simulink model "Controller_Simulation"  (R2025b)
settings: Solver=VariableStepAuto  StartTime=0.0  StopTime=100  RelTol=1e-3
undefined symbols (not defined in the file): cg_structure, chi, DiscIntNeverNeededParam, ESC_mass_same, g, Kd, Ki, Kp, M, m_carriage_bracket_and_cart, m_counter, m_struct, miu_k, Motor_mass_small, N, prop_mass_small
libraries: simulink x3, slpidlib x1, SignalEditorBlockLib x1
settings Model: Creator=adity  LastModifiedBy=33248

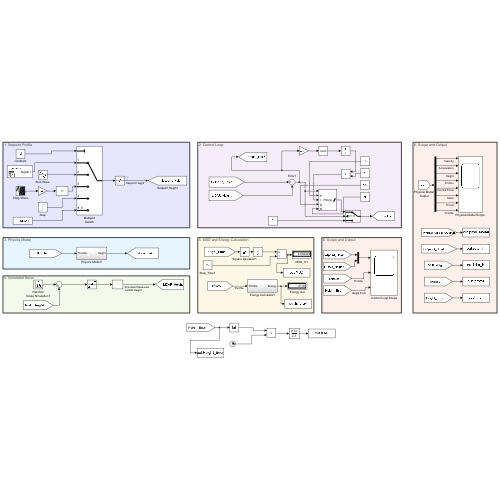
[thumbnail: Simulink's stored preview of the top-level diagram]
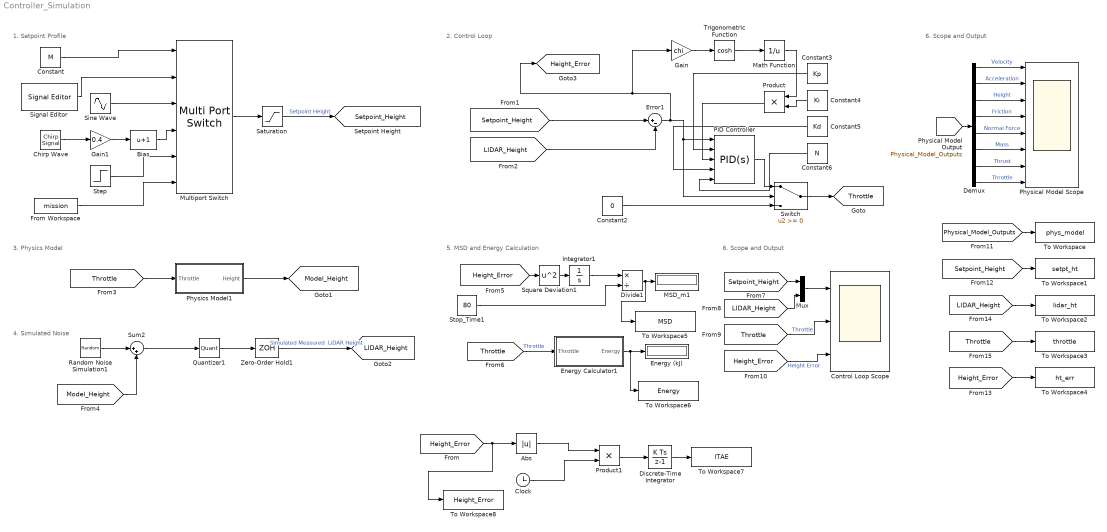
== system Controller_Simulation ==
  note: 6. Scope and Output
  note: 6. Scope and Output
  note: 5. MSD and Energy Calculation
  note: 4. Simulated Noise
  note: 3. Physics Model
  note: 2. Control Loop
  note: 1. Setpoint Profile
  Abs : Abs  SaturateOnIntegerOverflow=off
  Bias : Bias  Bias=1  SaturateOnIntegerOverflow=off
  Chirp Wave : simulink/Sources/Chirp Signal  f1=0.01  T=100  f2=0.5
  Clock : Clock
  Constant : Constant  Value=M
  Constant2 : Constant  Value=0
  Constant3 : Constant  Value=Kp
  Constant4 : Constant  Value=Ki
  Constant5 : Constant  Value=Kd
  Constant6 : Constant  Value=N
  Control Loop Scope : Scope  NumInputPorts=3
      settings: ActiveDisplayYMinimum=-0.74940462387190931  ActiveDisplayYMaximum=2.1498858123443716  DataLoggingVariableName=ScopeData2
  Demux : Demux  Outputs=8
  Discrete-Time Integrator : DiscreteIntegrator  SampleTime=-1  ICPrevOutput=DiscIntNeverNeededParam  ICPrevScaledInput=DiscIntNeverNeededParam
  Divide1 : Product  Inputs=*/
  Energy (kJ) : Display
  Energy Calculator1 : Subsystem
  Error1 : Sum  Inputs=|+-
  From Workspace : FromWorkspace  VariableName=mission
  Gain : Gain  Gain=chi
  Gain1 : Gain  Gain=0.4
  Integrator1 : Integrator
  MSD_m1 : Display
  Math Function : Math  Operator=reciprocal
  Multiport Switch : MultiPortSwitch  Inputs=5  SaturateOnIntegerOverflow=off  InputSameDT=off
  Mux : Mux  Inputs=2
  PID Controller : slpidlib/PID Controller  Controller=PID  Form=Parallel  TimeDomain=Continuous-time  UseExternalTs=off  SampleTime=-1  IntegratorMethod=Forward Euler  FilterMethod=Forward Euler  ControllerParametersSource=external  P=230  I=75  UseKiTs=off  D=50  UseExternalDerivativeSource=off  N=10  UseFilter=on  TunerSelectOption=Transfer Function Based (PID Tuner App)  InitialConditionSource=internal  InitialConditionForIntegrator=0  InitialConditionForFilter=0  DifferentiatorICPrevScaledInput=0  ExternalReset=none  TrackingMode=off  Kt=1  LimitOutput=on  SatLimitsSource=internal  UpperSaturationLimit=79.0425  LowerSaturationLimit=0  LinearizeAsGain=on  AntiWindupMode=clamping  Kb=1  LimitIntegrator=off  UpperIntegratorSaturationLimit=inf  LowerIntegratorSaturationLimit=-inf  POutMin=[]  POutMax=[]  IOutMin=[]  IOutMax=[]  DOutMin=[]  DOutMax=[]  NOutMin=[]  NOutMax=[]  SumOutMin=[]  SumOutMax=[]  SaturationOutMin=[]  SaturationOutMax=[]  PParamMin=[]  PParamMax=[]  IParamMin=[]  IParamMax=[]  DParamMin=[]  DParamMax=[]  NParamMin=[]  NParamMax=[]  KbParamMin=[]  KbParamMax=[]  KtParamMin=[]  KtParamMax=[]  KbOutMin=[]  KbOutMax=[]  KtOutMin=[]  KtOutMax=[]  IntegratorOutMin=[]  IntegratorOutMax=[]  FilterOutMin=[]  FilterOutMax=[]  SumI1OutMin=[]  SumI1OutMax=[]  SumI2OutMin=[]  SumI2OutMax=[]  SumI3OutMin=[]  SumI3OutMax=[]  SumI4OutMin=[]  SumI4OutMax=[]  SumDOutMin=[]  SumDOutMax=[]  DifferentiatorOutMin=[]  DifferentiatorOutMax=[]  FilterDiffOutCoefMin=[]  FilterDiffOutCoefMax=[]  ReciprocalOutMin=[]  ReciprocalOutMax=[]  SumDenOutMin=[]  SumDenOutMax=[]  SumNumOutMin=[]  SumNumOutMax=[]  DivideOutMin=[]  DivideOutMax=[]  UdiffTsProdOutMin=[]  UdiffTsProdOutMax=[]  NTsProdOutMin=[]  NTsProdOutMax=[]  UintegralTsProdOutMin=[]  UintegralTsProdOutMax=[]  UngainTsProdOutMin=[]  UngainTsProdOutMax=[]  ClampingZeroOutDataTypeStr=Inherit: Inherit via back propagation  ClampingZeroOutMin=[]  ClampingZeroOutMax=[]  FilterDenConstantOutDataTypeStr=Inherit: Inherit via back propagation  FilterDenConstantOutMin=[]  FilterDenConstantOutMax=[]  PCopyOutDataTypeStr=Inherit: Inherit via back propagation  PCopyOutMin=[]  PCopyOutMax=[]  NCopyOutDataTypeStr=Inherit: Inherit via back propagation  NCopyOutMin=[]  NCopyOutMax=[]  IntegratorContinuousStateAttributes=''  IntegratorStateMustResolveToSignalObject=off  IntegratorRTWStateStorageClass=Auto  FilterContinuousStateAttributes=''  FilterStateMustResolveToSignalObject=off  FilterRTWStateStorageClass=Auto  ParallelPVariant=ExternalParameters  IdealPVariant=Disabled  IVariant=ExternalParameters  DVariant=ExternalParameters  IntegratorVariant=Continuous  SatVariant=Enabled  AWVariant=ContClampingParallel  PCopyVariant=Disabled  TRVariant=Disabled  FdbkBlocksVariant=Forward  IdealPFdbkVariant=Disabled  SatFdbkVariant=Disabled  DerivativeFilterVariant=ContFilter  NVariant=ExternalParameters  NCopyVariant=Disabled  FilterICVariant=InternalICsFilter  IntegratorICVariant=InternalICs  ExternalResetVariant=Disabled  TRSumVariant=Passthrough  SumFdbkVariant=Disabled  SumVariant=Sum_PID  TsampFilterVariant=InternalTs  TsampNgainVariant=Passthrough  TsampIntegralVariant=Disabled_SignalSpec  ExternalSaturationOutDataTypeStr=Inherit: Same as second input  DerivativeSourceVariant=ErrorSignal  PreIntVariant=InternalPreInt
  Physical Model Scope : Scope  NumInputPorts=8
      settings: ActiveDisplayYMinimum=0.51277748941499457  ActiveDisplayYMaximum=1.1096551033755411  DataLoggingVariableName=ScopeData3
  Physics Model1 : Subsystem
  Product : Product
  Product1 : Product
  Quantizer1 : Quantizer  QuantizationInterval=0.001
  Random Noise Simulation1 : RandomNumber  Variance=5e-05  SampleTime=0.05
  Saturation : Saturate  UpperLimit=1.44  LowerLimit=0
  Signal Editor : SignalEditorBlockLib/Signal Editor  FileName=samplemission.mat  ActiveScenario=Scenario  ActiveSignal=Signal 1  IsBus=off  OutputBusObjectStr=Bus: BusObject  SampleTime=0  ZeroCross=off  OutputAfterFinalValue=Setting to zero  Unit=inherit  PreserveSignalName=on  ApplySigPropsToAllScenarios=on  ApplySigPropsToAllSignals=off  SignalPropertySource=Dialog parameters
  Sine Wave : Sin  Amplitude=1.44  SampleTime=0
  Square Deviation1 : Math  Operator=square
  Step : Step  Time=20  After=1.3  SampleTime=0
  Stop_Time1 : Constant  Value=80
  Sum2 : Sum  Inputs=|++
  Switch : Switch  SaturateOnIntegerOverflow=off  InputSameDT=off
  To Workspace : ToWorkspace  VariableName=phys_model  SaveFormat=Timeseries  SampleTime=-1
  To Workspace1 : ToWorkspace  VariableName=setpt_ht  SaveFormat=Timeseries  SampleTime=-1
  To Workspace2 : ToWorkspace  VariableName=lidar_ht  SaveFormat=Timeseries  SampleTime=-1
  To Workspace3 : ToWorkspace  VariableName=throttle  SaveFormat=Timeseries  SampleTime=-1
  To Workspace4 : ToWorkspace  VariableName=ht_err  SaveFormat=Timeseries  SampleTime=-1
  To Workspace5 : ToWorkspace  VariableName=MSD  SaveFormat=Timeseries  SampleTime=-1
  To Workspace6 : ToWorkspace  VariableName=Energy  SaveFormat=Timeseries  SampleTime=-1
  To Workspace7 : ToWorkspace  VariableName=ITAE  SaveFormat=Timeseries  SampleTime=-1
  To Workspace8 : ToWorkspace  VariableName=Height_Error  SaveFormat=Timeseries  SampleTime=-1
  Trigonometric Function : Trigonometry  Operator=cosh
  Zero-Order Hold1 : ZeroOrderHold  SampleTime=0.05
  tag scope: Height_Error=global, LIDAR_Height=global, Model_Height=global, Setpoint_Height=global, Throttle=global
  wires:
  Step/1 -> Multiport Switch/5
  Constant/1 -> Multiport Switch/1
  Multiport Switch/1 -> Saturation/1
  Saturation/1 -> [Setpoint_Height]  "Setpoint Height"
  Sine Wave/1 -> Multiport Switch/3
  [LIDAR_Height] -> Error1/2
  PID Controller/1 -> Switch/1
  Constant2/1 -> Switch/3
  Switch/1 -> [Throttle]
  [Setpoint_Height] -> Error1/1
  [Throttle] -> Physics Model1/1(Throttle)
  Physics Model1/1(Height) -> [Model_Height]
  Random Noise Simulation1/1 -> Sum2/1
  [Model_Height] -> Sum2/2
  Quantizer1/1 -> Zero-Order Hold1/1
  Sum2/1 -> Quantizer1/1
  Zero-Order Hold1/1 -> [LIDAR_Height]  "Simulated Measured  LiDAR Height"
  Integrator1/1 -> Divide1/1
  Divide1/1 -> To Workspace5/1, MSD_m1/1
  Stop_Time1/1 -> Divide1/2
  Square Deviation1/1 -> Integrator1/1
  [Height_Error] -> Square Deviation1/1
  [Throttle] -> Energy Calculator1/1(Throttle)  "Throttle"
  Energy Calculator1/1(Energy) -> To Workspace6/1, Energy (kJ)/1
  [Throttle] -> Control Loop Scope/2  "Throttle"
  [Height_Error] -> Control Loop Scope/3  "Height Error"
  [Physical_Model_Outputs] -> Demux/1
  Demux/1 -> Physical Model Scope/1  "Velocity"
  Demux/2 -> Physical Model Scope/2  "Acceleration"
  Demux/3 -> Physical Model Scope/3  "Height"
  Demux/4 -> Physical Model Scope/4  "Friction"
  Demux/5 -> Physical Model Scope/5  "Normal Force"
  Demux/6 -> Physical Model Scope/6  "Mass"
  Demux/7 -> Physical Model Scope/7  "Thrust"
  Demux/8 -> Physical Model Scope/8  "Throttle"
  [Physical_Model_Outputs] -> To Workspace/1
  [Setpoint_Height] -> To Workspace1/1
  [LIDAR_Height] -> To Workspace2/1
  [Height_Error] -> To Workspace4/1
  [Throttle] -> To Workspace3/1
  [Setpoint_Height] -> Mux/1
  [LIDAR_Height] -> Mux/2
  Mux/1 -> Control Loop Scope/1
  Constant3/1 -> PID Controller/2
  Constant5/1 -> PID Controller/4
  Constant6/1 -> PID Controller/5
  Error1/1 -> Gain/1, [Height_Error], Switch/2, PID Controller/1
  Gain/1 -> Trigonometric Function/1
  Trigonometric Function/1 -> Math Function/1
  Math Function/1 -> Product/1
  Constant4/1 -> Product/2
  Product/1 -> PID Controller/3
  Bias/1 -> Multiport Switch/4
  Chirp Wave/1 -> Gain1/1
  Gain1/1 -> Bias/1
  Signal Editor/1 -> Multiport Switch/2
  [Height_Error] -> To Workspace8/1, Abs/1
  Abs/1 -> Product1/1
  Clock/1 -> Product1/2
  Product1/1 -> Discrete-Time Integrator/1
  Discrete-Time Integrator/1 -> To Workspace7/1
  From Workspace/1 -> Multiport Switch/6

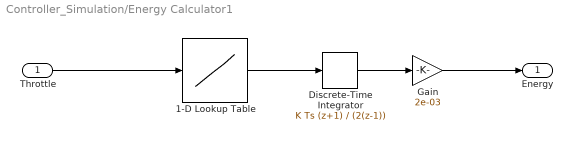
== system Controller_Simulation/Energy Calculator1 ==
  Throttle : Inport
  1-D Lookup Table : Lookup_n-D  NumberOfTableDimensions=1  BreakpointsForDimension1=[0.0, 0.0175925, 1.2377142, 3.1365067, 4.901275, 6.8963, 8.8838683, 10.9670175, 13.0595992, 14.9176417, 16.9770608, 18.969235, 21.1009383, 23.2400917, 25.325135, 27.58627, 29.690315, 31.6848525, 33.699295, 35.8387717, 37.8426708, 39.8378983, 42.0125808, 43.9547767, 46.0743067, 48.1062525, 50.1084, 52.1281567, 54.0838633, 56.1470767, 58.2021283, 60.3576092, 62.4913117, 64.523785, 66.5985917, 68.6827833, 70.7331533, 72.9931517, 74.9545758, 76.920765, 79.04246, 81.0915575, 83.0196342, 85.1594475, 87.4621408, 89.5253725, 91.7213858, 93.7960275, 95.8424125, 98.0918267, 99.8837325, 100.0]  Table=[0.59298494, 0.573685995, 0.495724685, 3.255271459, 9.483846138, 14.2184236, 19.52664974, 25.72707715, 32.50936139, 38.24910897, 45.0793771, 51.72372472, 56.42688246, 60.49341795, 73.2855129, 80.83023918, 87.08334294, 94.20105816, 100.0822784, 106.322355, 112.1062732, 117.9940577, 123.9954805, 128.5803796, 133.772233, 138.749002, 143.7563082, 147.707891, 151.8210984, 155.4051911, 158.9103922, 163.3354258, 166.8562986, 170.7617364, 174.5250378, 177.2673813, 181.5344629, 188.5850075, 197.7836109, 213.5394979, 223.7868027, 224.3463525, 224.5630136, 224.384079, 224.1956007, 224.1136788, 223.659762, 223.8476511, 223.5645398, 223.1671014, 223.0042697, 222.97161]  InterpMethod=Linear Lagrange  InternalRulePriority=Speed  RndMeth=Simplest
  Discrete-Time Integrator : DiscreteIntegrator  IntegratorMethod=Integration: Trapezoidal  SampleTime=0.05  RndMeth=Ceiling  ICPrevOutput=DiscIntNeverNeededParam  ICPrevScaledInput=DiscIntNeverNeededParam
  Gain : Gain  Gain=2e-03
  Energy : Outport
  wires:
  Throttle/1 -> 1-D Lookup Table/1
  Discrete-Time Integrator/1 -> Gain/1
  1-D Lookup Table/1 -> Discrete-Time Integrator/1
  Gain/1 -> Energy/1

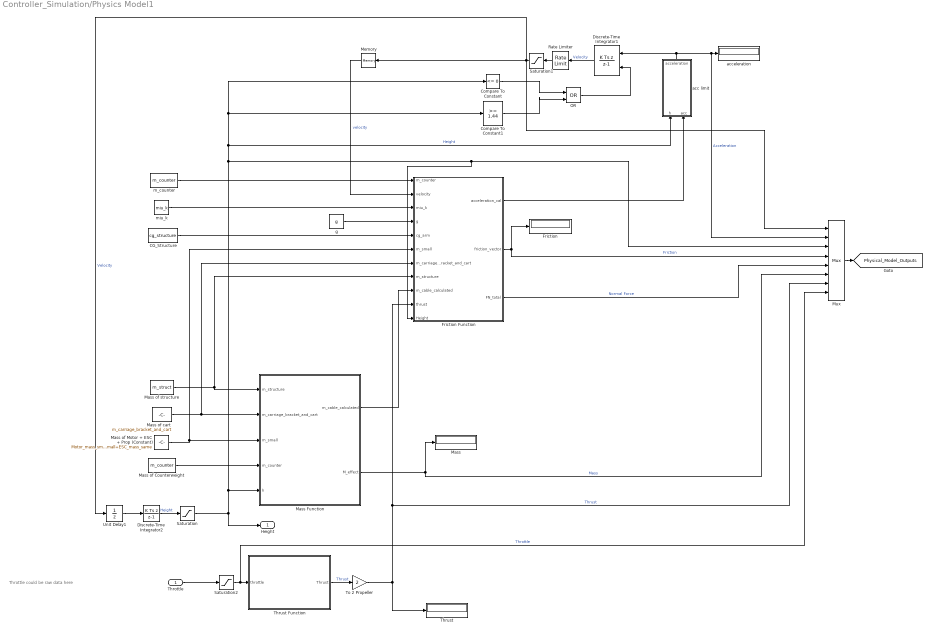
== system Controller_Simulation/Physics Model1 ==
  note: Throttle could be raw data here
  Throttle : Inport
  CG_Structure : Constant  Value=cg_structure
  Compare To Constant : simulink/Logic and Bit Operations/Compare To Constant  relop=<=  const=0  OutDataTypeStr=boolean
  Compare To Constant1 : simulink/Logic and Bit Operations/Compare To Constant  relop=>=  const=1.44  OutDataTypeStr=boolean
  Discrete-Time Integrator1 : DiscreteIntegrator  IntegratorMethod=Integration: Backward Euler  ExternalReset=rising  SampleTime=0.05  ICPrevOutput=DiscIntNeverNeededParam  ICPrevScaledInput=DiscIntNeverNeededParam
  Discrete-Time Integrator2 : DiscreteIntegrator  IntegratorMethod=Integration: Backward Euler  SampleTime=0.05  ICPrevOutput=DiscIntNeverNeededParam  ICPrevScaledInput=DiscIntNeverNeededParam
  Friction : Display
  Friction Function : MATLAB Function  TreatAsAtomicUnit=on
  Mass : Display
  Mass Function : MATLAB Function  TreatAsAtomicUnit=on
  Mass of Counterweight : Constant  Value=m_counter
  Mass of Motor + ESC + Prop (Constant) : Constant  Value=Motor_mass_small+prop_mass_small+ESC_mass_same
  Mass of cart : Constant  Value=m_carriage_bracket_and_cart
  Mass of structure : Constant  Value=m_struct
  Memory : Memory
  Mux : Mux  Inputs=8
  OR : Logic  Operator=OR  IconShape=distinctive  AllPortsSameDT=off  OutDataTypeStr=boolean
  Rate Limiter : RateLimiter  RisingSlewLimit=200  FallingSlewLimit=-200  SampleTimeMode=inherited
  Saturation : Saturate  UpperLimit=1.44  LowerLimit=0
  Saturation1 : Saturate  UpperLimit=15  LowerLimit=-15
  Saturation2 : Saturate  UpperLimit=100  LowerLimit=0
  Thrust : Display
  Thrust Function : MATLAB Function  TreatAsAtomicUnit=on
  To 2 Propeller : Gain  Gain=2
  Unit Delay1 : UnitDelay  SampleTime=0.05  HasFrameUpgradeWarning=on
  acc limit : MATLAB Function  TreatAsAtomicUnit=on
  acceleration : Display
  g : Constant  Value=g
  m_counter : Constant  Value=m_counter
  miu_k : Constant  Value=miu_k
  Height : Outport
  tag scope: Physical_Model_Outputs=global
  wires:
  miu_k/1 -> Friction Function/3(miu_k)
  acc limit/1(acceleration) -> Discrete-Time Integrator1/1, Mux/2, acceleration/1  "Acceleration"
  Saturation/1 -> Friction Function/11(Height), Mux/3, Compare To Constant/1, Compare To Constant1/1, acc limit/1(h), Mass Function/5(h), Height/1  "Height"
  Friction Function/1(acceleration_cal) -> acc limit/2(acc)
  Mass of cart/1 -> Mass Function/2(m_carriage_bracket_and_cart), Friction Function/7(m_carriage_bracket_and_cart)
  Friction Function/3(FN_total) -> Mux/5  "Normal Force"
  Unit Delay1/1 -> Discrete-Time Integrator2/1
  OR/1 -> Discrete-Time Integrator1/2
  Discrete-Time Integrator1/1 -> Rate Limiter/1  "Velocity"
  Mass of structure/1 -> Mass Function/1(m_structure), Friction Function/8(m_structure)
  Discrete-Time Integrator2/1 -> Saturation/1  "Height"
  Thrust Function/1(Thrust) -> To 2 Propeller/1  "Thrust"
  Memory/1 -> Friction Function/2(velocity)  "velocity"
  Mass of Counterweight/1 -> Mass Function/4(m_counter)
  g/1 -> Friction Function/4(g)
  Friction Function/2(friction_vector) -> Friction/1, Mux/4  "Friction"
  Compare To Constant/1 -> OR/1
  Mass Function/2(M_effect) -> Mux/6, Mass/1  "Mass"
  Rate Limiter/1 -> Saturation1/1
  CG_Structure/1 -> Friction Function/5(cg_arm)
  To 2 Propeller/1 -> Mux/7, Friction Function/10(thrust), Thrust/1  "Thrust"
  Saturation2/1 -> Mux/8, Thrust Function/1(throttle)  "Throttle"
  m_counter/1 -> Friction Function/1(m_counter)
  Mass Function/1(m_cable_calculated) -> Friction Function/9(m_cable_calculated)
  Compare To Constant1/1 -> OR/2
  Saturation1/1 -> Mux/1, Unit Delay1/1, Memory/1  "Velocity"
  Mass of Motor + ESC + Prop (Constant)/1 -> Mass Function/3(m_small), Friction Function/6(m_small)
  Throttle/1 -> Saturation2/1
  Mux/1 -> [Physical_Model_Outputs]

== matlab function Controller_Simulation/Physics Model1/Friction Function ==
  data: m_counter input; velocity input; miu_k input; g input; cg_arm input; m_small input; m_carriage_bracket_and_cart input; m_structure input; m_cable_calculated input; thrust input; acceleration_cal output; friction_vector output; FN_total output; Height input
function [acceleration_cal, friction_vector, FN_total] = friction_cal(m_counter, velocity, miu_k, g, cg_arm, m_small, m_carriage_bracket_and_cart, m_structure, m_cable_calculated, thrust, Height)
    %% Geometry & constants
    y_pad = 0.171; % measured on the carriage bracket model 

    F_static = 1.2753; % maximum F_static of ~130 g to each track
    F_static_ctr = F_static; % identical track

    % Centre of gravity / force, measured or calculated values
    cg_motor = 0.4225; % calculated using the CAD and measurements 
    x_thrust = cg_motor; % thrust assumed to act on cg_motor
    cg_cart = 0.0035; % calculated through measurement in the lab
    x_cable = 0.05; % measured in-person in the lab, 5 cm
    cg_counter = cg_cart; % counter mass block assumed aligned with cart CG

    %% Total mass calculation
    m_total = m_structure + 2*m_small + m_carriage_bracket_and_cart + ...
              m_cable_calculated + m_counter;

    %% Net driving force calculation
    % Positive = upward.
    F_drive = thrust - ...
              (m_carriage_bracket_and_cart + 2*m_small + m_structure + ...
               m_cable_calculated - m_counter) * g;

    %% Normal forces
    FN_raw = (m_carriage_bracket_and_cart * g * cg_cart + ...
              2 * g * m_small * cg_motor + ...
              m_structure * g * cg_arm + ...
              m_cable_calculated * g * x_cable - ...
              thrust * x_thrust - ...
              m_counter * g * cg_counter) / y_pad;

    % For a two-sided rail/pad contact, sign means loaded side.
    FN_total = abs(FN_raw);

    %% Static friction limit
    F_static_total = F_static + F_static_ctr;

    %% Hard-stop contact logic
    % If the carriage is at the bottom/top and the drive force pushes it
    % further into the stop, the stop reaction carries the load. rail friction should not pretend to be the holding force.

    hMin = 0.0;
    hMax = 1.44;
    hTol = 1e-6;

    atBottom = Height <= hMin + hTol;
    atTop    = Height >= hMax - hTol;

    if atBottom && F_drive < 0
        friction_vector = 0;
        acceleration_cal = 0;
        return
    end

    if atTop && F_drive > 0
        friction_vector = 0;
        acceleration_cal = 0;
        return
    end

    %% Dynamic friction level
    friction_dynamic_total = FN_total * miu_k;

    %% Smooth friction parameters
    v_s = 0.2014; % Stribeck velocity
    v_t = 0.504;  % tanh smoothing velocity
    c_v = 0.429;  % viscous damping coefficient 

    %% Static friction / breakaway patch
    velocity_zero_tol = 0.005;

    if abs(velocity) < velocity_zero_tol

        if abs(F_drive) <= F_static_total
            % TRUE STATIC FRICTION:
            % Mid-rail, almost stationary, and drive force small enough for
            % static friction to hold the carriage.
            friction_vector = -F_drive;
            acceleration_cal = 0;
            return

        else
            % BREAKAWAY:
            % Drive force exceeds static friction, so friction is maxed.
            friction_vector = -F_static_total * sign(F_drive);
        end

    else
        %% Smooth sign function
        smooth_sign = tanh(velocity / v_t);

        %% Continuous Stribeck curve
        friction_coulomb = friction_dynamic_total + ...
            (F_static_total - friction_dynamic_total) * exp(-(abs(velocity)/v_s)^2);

        %% Add viscous damping
        friction_vector = -friction_coulomb * smooth_sign - c_v * velocity;
    end

    %% Net acceleration
    acceleration_cal = (F_drive + friction_vector) / m_total;
end

== matlab function Controller_Simulation/Physics Model1/Mass Function ==
  data: m_cable_calculated output; m_structure input; m_carriage_bracket_and_cart input; m_small input; m_counter input; M_effect output; h input
function [m_cable_calculated, M_effect]= mass_func(m_structure, m_carriage_bracket_and_cart, m_small, m_counter, h)
    m_cable_calculated = calculate_cable_mass(h);
    M  = (2 * m_small) + m_carriage_bracket_and_cart + m_structure + 2*m_cable_calculated;
    M_effect = M - m_counter;   % effective mass for weight calc
end
%%------------------------------------------------------------------------
function m_supported = calculate_cable_mass(h)
    % ------------------ Physical Constants ------------------------------
    m_total = 0.190;        % Total mass of the cable (kg)
    L_total = 1.0;          % Total length of the cable (m)
    y_anchor = 0.44;        % Height of the fixed anchor point (m)
    % The height of the attachment point on the cart
    y_cart = h - 0.1052;
    % The vertical distance between the moving cart and the fixed anchor
    delta_y = y_cart - y_anchor;
    if delta_y >= L_total
        % Fully Taut Upward
        % The cart is so high that the entire 1m cable is pulled straight up.
        % The cart supports the entire weight of the cable.
        m_supported = m_total;
  
    else
        % U-Shape
        % Calculate the length of the chain on the cart's side of the "U"
        L_supported = (delta_y + L_total) / 2;
        
        % Convert supported length to supported mass
        m_supported = m_total * (L_supported/ L_total) ;
    end
end

== matlab function Controller_Simulation/Physics Model1/Thrust Function ==
  data: throttle input; Thrust output
function Thrust = thrust_cal(throttle)

if throttle <= 79.0425

    Thrust = ... %confirmed correct one
        -1.02178722e-11 * throttle^7 + ...
         3.31547781e-09 * throttle^6 + ...
        -4.23315827e-07 * throttle^5 + ...
         2.75535168e-05 * throttle^4 + ...
        -9.84949443e-04 * throttle^3 + ...
         1.84147041e-02 * throttle^2 + ...
        -2.92219275e-02 * throttle + ...
         5.09621010e-02;
    

else

    Thrust = 7.4300463179;

end

end

== matlab function Controller_Simulation/Physics Model1/acc limit ==
  data: h input; acc input; acceleration output
function acceleration = acc_limit(h, acc)
if h<=0 
    acceleration = max(acc,0);
elseif h>= 1.44
    acceleration = min(acc,0);
else
    acceleration = acc;
end
